simulink model "LoopStructure_Analysismodel"  (R2020b)
settings: Solver=VariableStepAuto  StartTime=0.0  StopTime=10.0  RelTol=1e-3
libraries: simulink x1
settings Model: Creator=Administrator  LastModifiedBy=Administrator

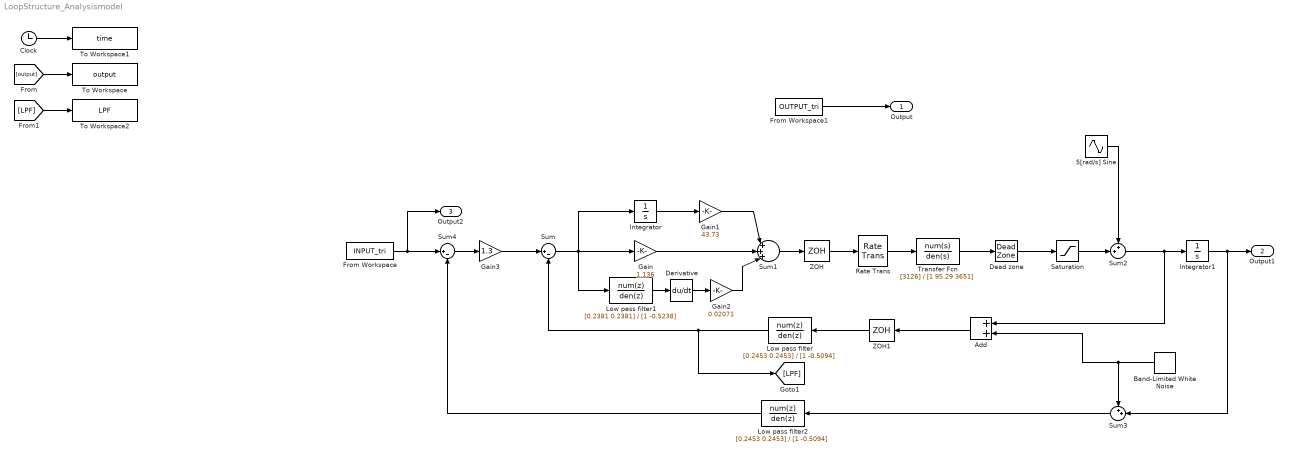
== system LoopStructure_Analysismodel ==
  5[rad/s] Sine : Sin  Amplitude=220  Frequency=5  SampleTime=0.005
  Add : Sum
  Band-Limited White Noise : simulink/Sources/Band-Limited White Noise  Cov=[0.000001]  Ts=0.005  seed=[52341]
  Clock : Clock
  Dead zone : DeadZone  LowerValue=2.5  UpperValue=2.5  SaturateOnIntegerOverflow=on
  Derivative : Derivative
  From Workspace : FromWorkspace  VariableName=INPUT_tri
  From Workspace1 : FromWorkspace  VariableName=OUTPUT_tri
  Gain : Gain  Gain=1.136
  Gain1 : Gain  Tag=z  Gain=43.73
  Gain2 : Gain  Gain=0.02071
  Gain3 : Gain  Gain=1.3
  Integrator : Integrator
  Integrator1 : Integrator
  Low pass filter : DiscreteTransferFcn  Numerator=[0.2453 0.2453]  Denominator=[1 -0.5094]  SampleTime=0.005
  Low pass filter1 : DiscreteTransferFcn  Numerator=[0.2381 0.2381]  Denominator=[1 -0.5238]  SampleTime=0.005
  Low pass filter2 : DiscreteTransferFcn  Numerator=[0.2453 0.2453]  Denominator=[1 -0.5094]  SampleTime=0.005
  Rate Trans : RateTransition  InitialCondition=0.005  OutPortSampleTime=0.005
  Saturation : Saturate  UpperLimit=300  LowerLimit=-300
  Sum : Sum  Inputs=|+-
  Sum1 : Sum  Inputs=|+++|
  Sum2 : Sum  Inputs=++|
  Sum3 : Sum  Inputs=++|
  Sum4 : Sum  Inputs=|+-
  To Workspace : ToWorkspace  VariableName=output  SampleTime=-1
  To Workspace1 : ToWorkspace  VariableName=time  SampleTime=-1
  To Workspace2 : ToWorkspace  VariableName=LPF  SaveFormat=Timeseries  SampleTime=-1
  Transfer Fcn : TransferFcn  Numerator=[3126]  Denominator=[1 95.29 3651]
  ZOH : ZeroOrderHold  SampleTime=0.005
  ZOH1 : ZeroOrderHold  SampleTime=0.005
  Output : Outport
  Output1 : Outport  Port=2
  Output2 : Outport  Port=3
  wires:
  [LPF] -> To Workspace2/1
  [output] -> To Workspace/1
  5[rad/s] Sine/1 -> Sum2/1
  Gain3/1 -> Sum/1
  Clock/1 -> To Workspace1/1
  ZOH/1 -> Rate Trans/1
  Rate Trans/1 -> Transfer Fcn/1
  Saturation/1 -> Sum2/2
  ZOH1/1 -> Low pass filter/1
  Low pass filter/1 -> [LPF], Sum/2
  Transfer Fcn/1 -> Dead zone/1
  Dead zone/1 -> Saturation/1
  Band-Limited White Noise/1 -> Sum3/1, Add/2
  Add/1 -> ZOH1/1
  Gain2/1 -> Sum1/3
  Derivative/1 -> Gain2/1
  Sum/1 -> Gain/1, Low pass filter1/1, Integrator/1
  Gain/1 -> Sum1/2
  Integrator/1 -> Gain1/1
  Gain1/1 -> Sum1/1
  Sum1/1 -> ZOH/1
  Low pass filter1/1 -> Derivative/1
  From Workspace1/1 -> Output/1
  From Workspace/1 -> Sum4/1, Output2/1
  Sum2/1 -> Add/1, Integrator1/1
  Integrator1/1 -> Output1/1, Sum3/2
  Sum3/1 -> Low pass filter2/1
  Sum4/1 -> Gain3/1
  Low pass filter2/1 -> Sum4/2
